simulink model "contfeedforwardr12"  (R2014b)
settings: Solver=ode15s  SolverMode=SingleTasking  StartTime=0.0  StopTime=10.0  RelTol=1e-3  AbsTol=1e-6
values from neighbouring files (symbols this model uses):
  dchange = [60, 150]    [run_sim_ol.m]    (also in run_sim_spec.m = sim_spec.dchange; singlenodescm2022.m = input('Enter the demand change [2000 units]: '))
  denqd = conv(conv(conv([lamd 1],[lamd 1]),[lamd 1]),[lamd 1])    [run_sim_spec.m]    (also in singlenodescm2022.m)
  denqf = conv(conv([lamdf 1],[lamdf 1]),[lamdf 1])    [run_sim_spec.m]    (also in singlenodescm2022.m)
  denqr = conv([lamr 1],[lamr 1])    [run_sim_spec.m]    (also in singlenodescm2022.m)
  ffcase = 0    [run_sim_spec.m]    (also in singlenodescm2022.m)
  ffswitch = ffswitch_values(i_sim)    [run_sim_spec.m]    (also in singlenodescm2022.m = 1)
  numqd = conv(conv([thetaptilde 1],[1 0]),[4*lamd 1])    [run_sim_spec.m]    (also in singlenodescm2022.m)
  numqf = conv(numqf,[thetaptilde-thetadtilde 1])    [run_sim_spec.m]    (also in singlenodescm2022.m)
  numqr = conv([0 1],[1 0])    [run_sim_spec.m]    (also in singlenodescm2022.m)
  rchange = [10, 1000]    [run_sim_ol.m]    (also in run_sim_spec.m = sim_spec.rchange; singlenodescm2022.m = input('Enter the inventory setpoint [20000 units]: '))
  thetad = sim_spec.thetad    [run_sim_spec.m]    (also in singlenodescm2022.m = input('Enter the disturbance forecast horizon (thetaf) [20 t)
  thetadtilde = (thetad-thetas)    [run_sim_spec.m]    (also in singlenodescm2022.m)
  thetap = 10    [run_sim_ol.m]    (also in run_sim_spec.m = sim_spec.thetap; singlenodescm2022.m = input('Enter the production lead time (thetap) [10 time unit)
  thetaptilde = thetap    [run_sim_spec.m]    (also in singlenodescm2022.m)
  thetas = 2    [run_sim_ol.m]    (also in run_sim_spec.m = sim_spec.thetas; singlenodescm2022.m = input('Enter the supply stream delivery time (thetad) [2 tim)
  vard = [85, 1000]    [run_sim_ol.m]    (also in run_sim_spec.m = sim_spec.vard; singlenodescm2022.m = input('Enter the unforecasted demand variance (vard) [1000]:)
settings Model: Creator=derivera  LastModifiedBy=derivera
settings DataIOCC: LimitDataPoints=off  SignalLoggingSaveFormat=ModelDataLogs
settings OptimizationCC: BooleanDataType=off
settings DebuggingCC: SaveWithParameterizedLinksMsg=none  UnderspecifiedInitializationDetection=Classic  MergeDetectMultiDrivingBlocksExec=none  SignalResolutionControl=TryResolveAllWithWarning  SolverPrmCheckMsg=none  MultiTaskDSMMsg=warning  MultiTaskCondExecSysMsg=none  StrictBusMsg=None
settings HardwareCC: TargetUnknown=on
settings RTWCC: IncludeERTFirstTime=on
settings GRTTargetCC: CombineOutputUpdateFcns=off  GRTInterface=on

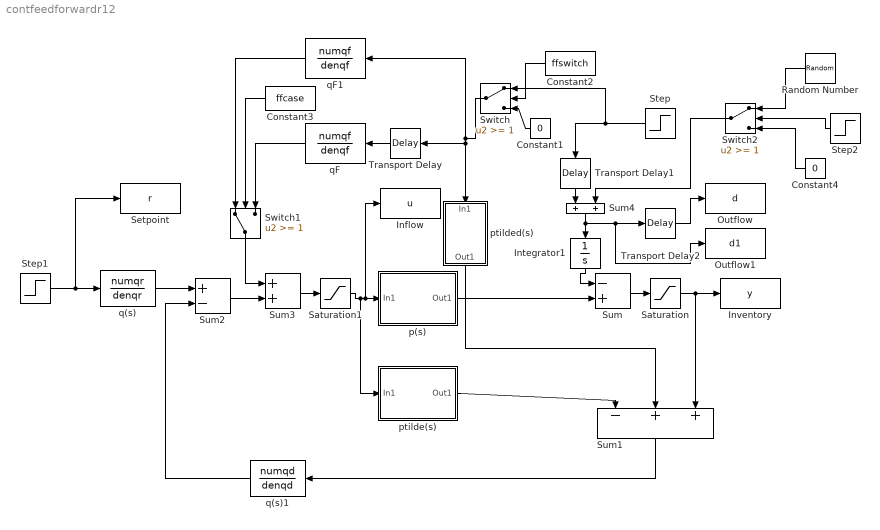
== system contfeedforwardr12 ==
  Constant1 : Constant  Value=0
  Constant2 : Constant  Value=ffswitch
  Constant3 : Constant  Value=ffcase
  Constant4 : Constant  Value=0
  Inflow : ToWorkspace  VariableName=u  SampleTime=-1
  Integrator1 : Integrator
  Inventory : ToWorkspace  VariableName=y  SampleTime=-1
  Outflow : ToWorkspace  VariableName=d  SampleTime=-1
  Outflow1 : ToWorkspace  VariableName=d1  SampleTime=-1
  Random Number : RandomNumber  Variance=vard  SampleTime=1
  Saturation : Saturate  UpperLimit=inf  LowerLimit=-inf
  Saturation1 : Saturate  UpperLimit=inf  LowerLimit=-inf
  Setpoint : ToWorkspace  VariableName=r  SampleTime=-1
  Step : Step  Time=50  After=dchange  SampleTime=0
  Step1 : Step  After=rchange  SampleTime=0
  Step2 : Step  Time=85  SampleTime=0
  Sum : Sum  Inputs=-+  SaturateOnIntegerOverflow=on  InputSameDT=on  OutDataTypeStr=Inherit: Same as first input
  Sum1 : Sum  Inputs=-++  SaturateOnIntegerOverflow=on  InputSameDT=on  OutDataTypeStr=Inherit: Same as first input
  Sum2 : Sum  Inputs=+-  SaturateOnIntegerOverflow=on  InputSameDT=on  OutDataTypeStr=Inherit: Same as first input
  Sum3 : Sum  SaturateOnIntegerOverflow=on  InputSameDT=on  OutDataTypeStr=Inherit: Same as first input
  Sum4 : Sum  SaturateOnIntegerOverflow=on  InputSameDT=on  OutDataTypeStr=Inherit: Same as first input
  Switch : Switch  Threshold=1  SaturateOnIntegerOverflow=on  InputSameDT=on
  Switch1 : Switch  Threshold=1  SaturateOnIntegerOverflow=on  InputSameDT=on
  Switch2 : Switch  Threshold=1  SaturateOnIntegerOverflow=on  InputSameDT=on
  Transport Delay : TransportDelay  DelayTime=max(thetadtilde-thetaptilde,0)
  Transport Delay1 : TransportDelay  DelayTime=(thetad-thetas)
  Transport Delay2 : TransportDelay  DelayTime=thetas
  p(s) : Subsystem
  ptilde(s) : Subsystem
  ptilded(s) : Subsystem
  q(s) : TransferFcn  Numerator=numqr  Denominator=denqr
  q(s)1 : TransferFcn  Numerator=numqd  Denominator=denqd
  qF : TransferFcn  Numerator=numqf  Denominator=denqf
  qF1 : TransferFcn  Numerator=numqf  Denominator=denqf
  wires:
  p(s)/1(Out1) -> Sum/2
  Integrator1/1 -> Sum/1
  ptilde(s)/1(Out1) -> Sum1/1
  ptilded(s)/1(Out1) -> Sum1/2
  Sum2/1 -> Sum3/2
  Sum1/1 -> q(s)1/1
  q(s)1/1 -> Sum2/2
  q(s)/1 -> Sum2/1
  Step1/1 -> q(s)/1, Setpoint/1
  Constant1/1 -> Switch/3
  Constant2/1 -> Switch/2
  Transport Delay/1 -> qF/1
  Switch1/1 -> Sum3/1
  qF/1 -> Switch1/3
  Switch/1 -> ptilded(s)/1(In1), Transport Delay/1, qF1/1
  qF1/1 -> Switch1/1
  Constant3/1 -> Switch1/2
  Sum/1 -> Saturation/1
  Saturation/1 -> Inventory/1, Sum1/3
  Sum3/1 -> Saturation1/1
  Saturation1/1 -> ptilde(s)/1(In1), p(s)/1(In1), Inflow/1
  Step/1 -> Transport Delay1/1, Switch/1
  Transport Delay2/1 -> Outflow/1
  Sum4/1 -> Integrator1/1, Transport Delay2/1, Outflow1/1
  Transport Delay1/1 -> Sum4/1
  Step2/1 -> Switch2/2
  Constant4/1 -> Switch2/3
  Switch2/1 -> Sum4/2
  Random Number/1 -> Switch2/1

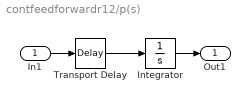
== system contfeedforwardr12/p(s) ==
  In1 : Inport
  Integrator : Integrator
  Transport Delay : TransportDelay  DelayTime=thetap
  Out1 : Outport  InitialOutput=0
  wires:
  Transport Delay/1 -> Integrator/1
  Integrator/1 -> Out1/1
  In1/1 -> Transport Delay/1

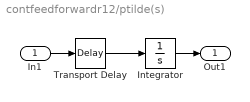
== system contfeedforwardr12/ptilde(s) ==
  In1 : Inport
  Integrator : Integrator
  Transport Delay : TransportDelay  DelayTime=thetaptilde
  Out1 : Outport  InitialOutput=0
  wires:
  Transport Delay/1 -> Integrator/1
  Integrator/1 -> Out1/1
  In1/1 -> Transport Delay/1

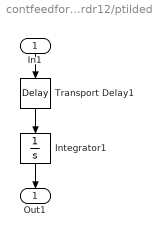
== system contfeedforwardr12/ptilded(s) ==
  In1 : Inport
  Integrator1 : Integrator
  Transport Delay1 : TransportDelay  DelayTime=thetadtilde
  Out1 : Outport  InitialOutput=0
  wires:
  Transport Delay1/1 -> Integrator1/1
  In1/1 -> Transport Delay1/1
  Integrator1/1 -> Out1/1
